simulink model "Cooperative_Quad_09_VelEst_02"  (R2017b)
settings: Solver=ode45  StartTime=0.0  StopTime=120  RelTol=1e-3  EnableMultiTasking=on
InitFcn:
  | Const_Vel_Est_02
values from neighbouring files (symbols this model uses):
  alpha = 1.0e-5    (= 1e-05)    [Cons_AMFC_Quad_New_01.m]    (also in Const_Vel_Est_02.m = 0.1; constant_Rev01_4Agents_10.m = 0.1; constant_Rev01_4Agents_9.m = 0.1)
  alpha_Slid = 0.01    [Cons_AMFC_Quad_New_01.m]    (also in Const_Vel_Est_02.m)
  AN = [     0 1 0 0 ... (first row only)    [Const_Vel_Est_02.m]    (also in constant_Rev01_4Agents_10.m; constant_Rev01_4Agents_9.m)
  B = 1e+0*eye(n)    [Cons_AMFC_Quad_New_01.m]    (also in Const_Vel_Est_02.m = 1e0*eye(n); constant_Rev01_4Agents_10.m = 1e0*eye(n); constant_Rev01_4Agents_9.m = 1e0*eye(n))
  BBT_inv = ((B'*B)^(-1))*B'    [Cons_AMFC_Quad_New_01.m]    (also in Const_Vel_Est_02.m; constant_Rev01_4Agents_10.m; constant_Rev01_4Agents_9.m)
  BN = [     1 0 0 0 ... (first row only)    [Const_Vel_Est_02.m]    (also in constant_Rev01_4Agents_10.m; constant_Rev01_4Agents_9.m)
  epsilon_struct = struct('data',epsilon_InitVal)    [Const_Vel_Est_02.m]    (also in constant_Rev01_4Agents_10.m; constant_Rev01_4Agents_9.m)
  g = 9.81    [Const_Vel_Est_02.m]    (also in Swing2d_01_const.m; constant_Rev01_4Agents_10.m; constant_Rev01_4Agents_9.m)
  gamma_0 = 1e-0*diag([1e-3*ones(3,1);1e-0*ones(3,1)])    [Cons_AMFC_Quad_New_01.m]    (also in Const_Vel_Est_02.m = 1e-1*diag([1e-3*ones(3,1);1e-0*ones(3,1)]); constant_Rev01_4Agents_10.m = 1e+1*diag([1e-3*ones(3,1);1e-0*ones(3,1)]); constant_Rev01_4Agents_9.m = 1e+1*diag([1e-3*ones(6,1);1e-0*ones(6,1)]))
  gamma_1 = 1e+2*diag([1e-3*ones(3,1);1e-0*ones(3,1)])    [Cons_AMFC_Quad_New_01.m]    (also in Const_Vel_Est_02.m; constant_Rev01_4Agents_10.m = 1e+3*diag([1e-3*ones(3,1);1e0*ones(3,1)]); constant_Rev01_4Agents_9.m = 1e+3*diag([1e-3*ones(6,1);1e0*ones(6,1)]))
  H = L + BN    [Const_Vel_Est_02.m]    (also in constant_Rev01_4Agents_10.m; constant_Rev01_4Agents_9.m)
  J = 1.2416e-3 * diag([1 1 2])    [Cons_AMFC_Quad_New_01.m]    (also in Const_Vel_Est_02.m = 1.2416e-3 * diag([1 1 2],0); constant_Rev01_4Agents_10.m = 1.2416e-3 * diag([1 1 2],0); constant_Rev01_4Agents_9.m = 1.2416e-3 * diag([1 1 2],0))
  k1 = 10    [Cons_AMFC_Quad_New_01.m]    (also in Const_Vel_Est_02.m = 1; constant_Rev01_4Agents_10.m = 1; constant_Rev01_4Agents_9.m = 1)
  k1o = 1000    [Cons_AMFC_Quad_New_01.m]    (also in Const_Vel_Est_02.m)
  k2 = 0.1    [Cons_AMFC_Quad_New_01.m]    (also in Const_Vel_Est_02.m; constant_Rev01_4Agents_10.m = 1; constant_Rev01_4Agents_9.m = 1)
  k2o = 100    [Cons_AMFC_Quad_New_01.m]    (also in Const_Vel_Est_02.m)
  Ka = 0.01    [Cons_AMFC_Quad_New_01.m]    (also in Const_Vel_Est_02.m; constant_Rev01_4Agents_10.m; constant_Rev01_4Agents_9.m)
  Kd = 0.01    [Cons_AMFC_Quad_New_01.m]    (also in Const_Vel_Est_02.m; constant_Rev01_4Agents_10.m; constant_Rev01_4Agents_9.m)
  Kf = 1.0e-5    (= 1e-05)    [Cons_AMFC_Quad_New_01.m]    (also in Const_Vel_Est_02.m; constant_Rev01_4Agents_10.m; constant_Rev01_4Agents_9.m)
  Kt = 0.0435 * Kf    (= 4.35e-07)    [Cons_AMFC_Quad_New_01.m]    (also in Const_Vel_Est_02.m = 1e-07; constant_Rev01_4Agents_10.m = 1e-07; constant_Rev01_4Agents_9.m = 1e-07)
  Lq = 0.2    [Const_Vel_Est_02.m]    (also in constant_Rev01_4Agents_10.m; constant_Rev01_4Agents_9.m)
  m = 6    [Cons_AMFC_Quad_New_01.m]    (also in Const_Vel_Est_02.m; Swing2d_01_const.m = 1)
  M = 2.95    [Cons_AMFC_Quad_New_01.m]    (also in Const_Vel_Est_02.m = 2; constant_Rev01_4Agents_10.m = 2; constant_Rev01_4Agents_9.m = 2)
  Mb_P = Mb_val_P*ones(np,1)    [Const_Vel_Est_02.m]
  Mb_V = Mb_val_V*ones(np,1)    [Const_Vel_Est_02.m]
  Mu_P = 10    [Const_Vel_Est_02.m]
  Mu_V = 10    [Const_Vel_Est_02.m]
  n = 6    [Cons_AMFC_Quad_New_01.m]    (also in Const_Vel_Est_02.m; constant_Rev01_4Agents_10.m; constant_Rev01_4Agents_9.m = 12)
  N = 4    [Const_Vel_Est_02.m]    (also in constant_Rev01_4Agents_10.m; constant_Rev01_4Agents_9.m)
  n0 = 3    [Const_Vel_Est_02.m]    (also in constant_Rev01_4Agents_10.m; constant_Rev01_4Agents_9.m)
  np = 2    [Const_Vel_Est_02.m]
  Observer_Gain = 100    [Const_Vel_Est_02.m]    (also in constant_Rev01_4Agents_10.m; constant_Rev01_4Agents_9.m)
  Observer_Gain1 = 100    [Const_Vel_Est_02.m]    (also in constant_Rev01_4Agents_10.m = 10; constant_Rev01_4Agents_9.m = 10)
  Q = 1e-1*eye(n)    [Cons_AMFC_Quad_New_01.m]    (also in Const_Vel_Est_02.m = 1e-2*eye(n); constant_Rev01_4Agents_10.m = 1e-3*eye(n); constant_Rev01_4Agents_9.m = 1e-3*eye(n))
  R = 1e+0*eye(m)    [Cons_AMFC_Quad_New_01.m]    (also in Const_Vel_Est_02.m = 1e-0*eye(n); constant_Rev01_4Agents_10.m = 1e-0*eye(n); constant_Rev01_4Agents_9.m = 1e-0*eye(n))
  rho_0 = 1e-1    (= 0.1)    [Cons_AMFC_Quad_New_01.m]    (also in Const_Vel_Est_02.m; constant_Rev01_4Agents_10.m = 10; constant_Rev01_4Agents_9.m = 10)
  rho_1 = 1e-0    (= 1)    [Cons_AMFC_Quad_New_01.m]    (also in Const_Vel_Est_02.m; constant_Rev01_4Agents_10.m = 0.1; constant_Rev01_4Agents_9.m = 0.1)
  T_struct = struct('data',T_InitVal)    [Const_Vel_Est_02.m]    (also in constant_Rev01_4Agents_10.m; constant_Rev01_4Agents_9.m)
  U_dot0_M = U_dot0_m*ones(n0,1)    [Const_Vel_Est_02.m]    (also in constant_Rev01_4Agents_10.m; constant_Rev01_4Agents_9.m)
  Upsilon_M = Upsilon_m*ones(n0,1)    [Const_Vel_Est_02.m]    (also in constant_Rev01_4Agents_10.m; constant_Rev01_4Agents_9.m)
undefined symbols (not defined in the file or in its folder): sigbuilder_block
(part 1 of 5)
settings Model: SimulationMode=rapid-accelerator  Creator=hp  LastModifiedBy=ali.safaei
settings DataIOCC: LimitDataPoints=on  SaveFormat=Array
settings OptimizationCC: LifeSpan=inf
settings DebuggingCC: UnderspecifiedInitializationDetection=Classic  MergeDetectMultiDrivingBlocksExec=none  SFUnexpectedBacktrackingDiag=warning  SFNoUnconditionalDefaultTransitionDiag=warning  SFExecutionAtInitializationDiag=none
settings HardwareCC: ProdBitPerPointer=32  ProdBitPerSizeT=32  ProdBitPerPtrDiffT=32  ProdLargestAtomicFloat=None  ProdIntDivRoundTo=Undefined  ProdEndianess=Unspecified  ProdWordSize=32  ProdHWDeviceType=32-bit Generic
settings ModelReferenceCC: PropagateSignalLabelsOutOfModel=off
settings CodeAppCC: StateflowObjectComments=on
settings GRTTargetCC: TargetLangStandard=C89/C90 (ANSI)  GeneratePreprocessorConditionals=Disable all
settings ConfigComp: CovMetricSettings=dw  CovHtmlReporting=on  CovSaveCumulativeToWorkspaceVar=on  CovSaveSingleToWorkspaceVar=on  CovExternalEMLEnable=off

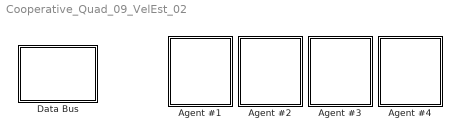
== system Cooperative_Quad_09_VelEst_02 ==
  Agent #1 : Subsystem
  Agent #2 : Subsystem
  Agent #3 : Subsystem
  Agent #4 : Subsystem
  "Data Bus " : Subsystem

== system Cooperative_Quad_09_VelEst_02/Agent #1 ==
  Agent # : Constant
  Constant1 : Constant  Value=zeros(2,1)
  Constant2 : Constant  Value=zeros(2,1)
  Decenteralized Cooperaive Controller #1 : Subsystem
  Mux1 : Mux
  Mux2 : Mux
  Plant #1 : Subsystem
  Relative estimations-1 : Subsystem
  tag scope: Acc1_XY=global, P_rel01_XY=global, P_rel1_XY=global, Pos1_XY=global, Pos1_Z=global, V_rel01_XY=global, V_rel1_XY=global, Vel1_XY=global, x1=global
  wires:
  Agent #/1 -> Decenteralized Cooperaive Controller #1/1(Agent #)
  Plant #1/1(X) -> [x1]
  Decenteralized Cooperaive Controller #1/1(u1) -> Plant #1/1(U)
  Plant #1/2(P_XY) -> Relative estimations-1/1(P_local_XY), [Pos1_XY]
  Plant #1/3(A_XY) -> [Acc1_XY], Relative estimations-1/2(A_local_XY)
  Mux1/1 -> [P_rel1_XY]
  Relative estimations-1/7(P10_est) -> [P_rel01_XY]
  Constant2/1 -> Mux1/1
  Relative estimations-1/8(V10_est) -> [V_rel01_XY]
  Constant1/1 -> Mux2/1
  Mux2/1 -> [V_rel1_XY]
  Relative estimations-1/1(P12_est) -> Mux1/2
  Relative estimations-1/3(P13_est) -> Mux1/3
  Relative estimations-1/5(P14_est) -> Mux1/4
  Relative estimations-1/2(V12_est) -> Mux2/2
  Relative estimations-1/4(V13_est) -> Mux2/3
  Relative estimations-1/6(V14_est) -> Mux2/4
  Plant #1/4(P_Z) -> [Pos1_Z]
  Plant #1/5(V_XY) -> [Vel1_XY]

== system Cooperative_Quad_09_VelEst_02/Agent #2 ==
  Agent # : Constant  Value=2
  Constant1 : Constant  Value=zeros(2,1)
  Constant2 : Constant  Value=zeros(2,1)
  Decenteralized Cooperaive Controller #2 : Subsystem
  Mux1 : Mux
  Mux2 : Mux
  Plant #2 : Subsystem
  Relative estimations-2 : Subsystem
  tag scope: Acc2_XY=global, P_rel02_XY=global, P_rel2_XY=global, Pos2_XY=global, Pos2_Z=global, V_rel02_XY=global, V_rel2_XY=global, Vel2_XY=global, x2=global
  wires:
  Plant #2/4(P_Z) -> [Pos2_Z]
  Relative estimations-2/6(V24_est) -> Mux2/4
  Relative estimations-2/4(V23_est) -> Mux2/3
  Relative estimations-2/2(V21_est) -> Mux2/2
  Relative estimations-2/5(P24_est) -> Mux1/4
  Relative estimations-2/3(P23_est) -> Mux1/3
  Relative estimations-2/1(P21_est) -> Mux1/2
  Mux2/1 -> [V_rel2_XY]
  Constant1/1 -> Mux2/1
  Relative estimations-2/8(V20_est) -> [V_rel02_XY]
  Constant2/1 -> Mux1/1
  Relative estimations-2/7(P20_est) -> [P_rel02_XY]
  Mux1/1 -> [P_rel2_XY]
  Plant #2/3(A_XY) -> [Acc2_XY], Relative estimations-2/2(A_local_XY)
  Plant #2/2(P_XY) -> [Pos2_XY], Relative estimations-2/1(P_local_XY)
  Decenteralized Cooperaive Controller #2/1(u2) -> Plant #2/1(U)
  Plant #2/1(X) -> [x2]
  Agent #/1 -> Decenteralized Cooperaive Controller #2/1(Agent #)
  Plant #2/5(V_XY) -> [Vel2_XY]

== system Cooperative_Quad_09_VelEst_02/Agent #3 ==
  Agent # : Constant  Value=3
  Constant1 : Constant  Value=zeros(2,1)
  Constant2 : Constant  Value=zeros(2,1)
  Decenteralized Cooperaive Controller #3 : Subsystem
  Mux1 : Mux
  Mux2 : Mux
  Plant #3 : Subsystem
  Relative estimations-3 : Subsystem
  tag scope: Acc3_XY=global, P_rel03_XY=global, P_rel3_XY=global, Pos3_XY=global, Pos3_Z=global, V_rel03_XY=global, V_rel3_XY=global, Vel3_XY=global, x3=global
  wires:
  Agent #/1 -> Decenteralized Cooperaive Controller #3/1(Agent #)
  Plant #3/1(X) -> [x3]
  Decenteralized Cooperaive Controller #3/1(u3) -> Plant #3/1(U)
  Plant #3/2(P_XY) -> Relative estimations-3/1(P_local_XY), [Pos3_XY]
  Plant #3/3(A_XY) -> [Acc3_XY], Relative estimations-3/2(A_local_XY)
  Mux1/1 -> [P_rel3_XY]
  Relative estimations-3/7(P30_est) -> [P_rel03_XY]
  Constant2/1 -> Mux1/1
  Relative estimations-3/8(V30_est) -> [V_rel03_XY]
  Constant1/1 -> Mux2/1
  Mux2/1 -> [V_rel3_XY]
  Relative estimations-3/1(P31_est) -> Mux1/2
  Relative estimations-3/3(P32_est) -> Mux1/3
  Relative estimations-3/5(P34_est) -> Mux1/4
  Relative estimations-3/2(V31_est) -> Mux2/2
  Relative estimations-3/4(V32_est) -> Mux2/3
  Relative estimations-3/6(V34_est) -> Mux2/4
  Plant #3/4(P_Z) -> [Pos3_Z]
  Plant #3/5(V_XY) -> [Vel3_XY]

== system Cooperative_Quad_09_VelEst_02/Agent #4 ==
  Agent # : Constant  Value=4
  Constant1 : Constant  Value=zeros(2,1)
  Constant2 : Constant  Value=zeros(2,1)
  Decenteralized Cooperaive Controller #4 : Subsystem
  Mux1 : Mux
  Mux2 : Mux
  Plant #4 : Subsystem
  Relative estimations-4 : Subsystem
  tag scope: Acc4_XY=global, P_rel04_XY=global, P_rel4_XY=global, Pos4_XY=global, Pos4_Z=global, V_rel04_XY=global, V_rel4_XY=global, Vel4_XY=global, x4=global
  wires:
  Plant #4/4(P_Z) -> [Pos4_Z]
  Relative estimations-4/6(V43_est) -> Mux2/4
  Relative estimations-4/4(V42_est) -> Mux2/3
  Relative estimations-4/2(V41_est) -> Mux2/2
  Relative estimations-4/5(P43_est) -> Mux1/4
  Relative estimations-4/3(P42_est) -> Mux1/3
  Relative estimations-4/1(P41_est) -> Mux1/2
  Mux2/1 -> [V_rel4_XY]
  Constant1/1 -> Mux2/1
  Relative estimations-4/8(V40_est) -> [V_rel04_XY]
  Constant2/1 -> Mux1/1
  Relative estimations-4/7(P40_est) -> [P_rel04_XY]
  Mux1/1 -> [P_rel4_XY]
  Plant #4/3(A_XY) -> Relative estimations-4/2(A_local_XY), [Acc4_XY]
  Plant #4/2(P_XY) -> Relative estimations-4/1(P_local_XY), [Pos4_XY]
  Decenteralized Cooperaive Controller #4/1(u4) -> Plant #4/1(U)
  Plant #4/1(X) -> [x4]
  Agent #/1 -> Decenteralized Cooperaive Controller #4/1(Agent #)
  Plant #4/5(V_XY) -> [Vel4_XY]

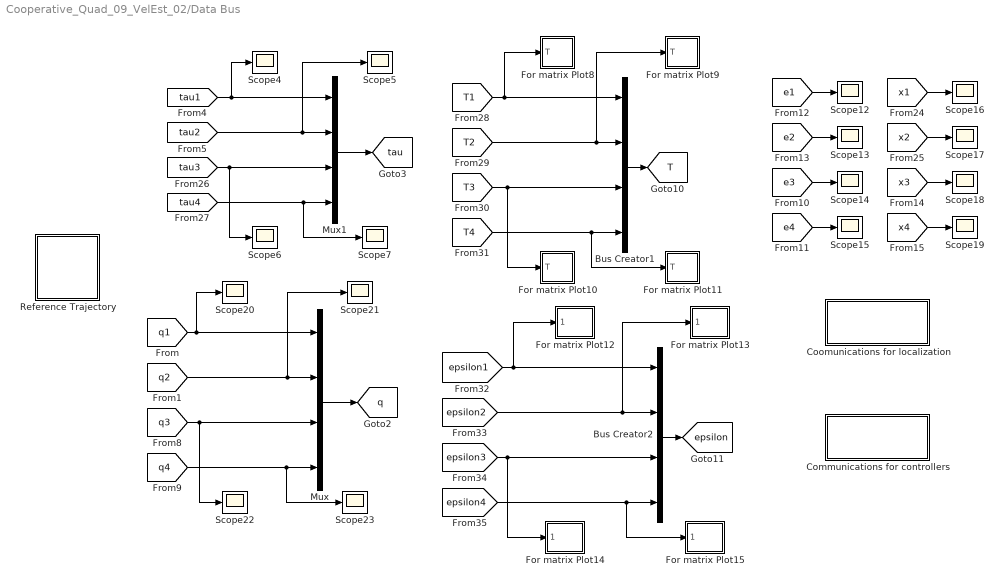
== system Cooperative_Quad_09_VelEst_02/Data Bus  ==
  Bus Creator1 : BusCreator  Inputs=4  OutDataTypeStr=Bus: T_bus
  Bus Creator2 : BusCreator  Inputs=4  OutDataTypeStr=Bus: epsilon_bus
  Communications for controllers : Subsystem
  Coomunications for localization : Subsystem
  For matrix Plot10 : Subsystem
  For matrix Plot11 : Subsystem
  For matrix Plot12 : Subsystem
  For matrix Plot13 : Subsystem
  For matrix Plot14 : Subsystem
  For matrix Plot15 : Subsystem
  For matrix Plot8 : Subsystem
  For matrix Plot9 : Subsystem
  Mux : Mux
  Mux1 : Mux
  Reference Trajectory : Subsystem
  Scope{4..7,12..23} (16 alike) : Scope
  tag scope: T=global, epsilon=global, q=global, tau=global
  wires:
  [q2] -> Scope21/1, Mux/2
  [tau1] -> Scope4/1, Mux1/1
  [tau2] -> Scope5/1, Mux1/2
  Mux1/1 -> [tau]
  [q1] -> Scope20/1, Mux/1
  Mux/1 -> [q]
  [e2] -> Scope13/1
  [e1] -> Scope12/1
  [x1] -> Scope16/1
  [q4] -> Scope23/1, Mux/4
  [q3] -> Scope22/1, Mux/3
  [e3] -> Scope14/1
  [e4] -> Scope15/1
  [x3] -> Scope18/1
  [x4] -> Scope19/1
  [tau3] -> Scope6/1, Mux1/3
  [tau4] -> Scope7/1, Mux1/4
  [T2] -> For matrix Plot9/1(T), Bus Creator1/2
  [T1] -> For matrix Plot8/1(T), Bus Creator1/1
  Bus Creator1/1 -> [T]
  [T3] -> For matrix Plot10/1(T), Bus Creator1/3
  [T4] -> For matrix Plot11/1(T), Bus Creator1/4
  [epsilon2] -> For matrix Plot13/1(epsilon), Bus Creator2/2
  [epsilon1] -> For matrix Plot12/1(epsilon), Bus Creator2/1
  Bus Creator2/1 -> [epsilon]
  [epsilon3] -> For matrix Plot14/1(epsilon), Bus Creator2/3
  [epsilon4] -> For matrix Plot15/1(epsilon), Bus Creator2/4
  [x2] -> Scope17/1

== system Cooperative_Quad_09_VelEst_02/Agent #1/Decenteralized Cooperaive Controller #1 ==
  Agent # : Inport
  Ali-1 : Subsystem
  "Computing xd-1 " : MATLAB Function  TreatAsAtomicUnit=on
  Cooperative Observers for X-1 : Subsystem
  Cooperative Observers for Xd-1 : Subsystem
  Mux : Mux  Inputs=2
  Subsystem : Subsystem
  Sum2 : Sum  Inputs=|+-
  u1 : Outport
  tag scope: e1=global
  wires:
  Agent #/1 -> "Computing xd-1 "/3(Agent_Num), Cooperative Observers for Xd-1/1(Agent No.), Cooperative Observers for X-1/1(Agent No.)
  Ali-1/1(u) -> u1/1
  "Computing xd-1 "/1(xd) -> Subsystem/1(In1)
  Subsystem/1(Out1) -> Sum2/1, Ali-1/2(xd)
  Cooperative Observers for Xd-1/1(q1) -> "Computing xd-1 "/1(q_i)
  Cooperative Observers for Xd-1/2(T1) -> "Computing xd-1 "/2(T_i)
  Cooperative Observers for X-1/1(X_est1) -> Ali-1/1(x)
  Sum2/1 -> [e1]
  [Pos1_XY] -> Mux/1
  Mux/1 -> Sum2/2
  [Pos1_Z] -> Mux/2

== system Cooperative_Quad_09_VelEst_02/Agent #1/Plant #1 ==
  U : Inport
  Clock : Clock
  Demux1 : Demux
  Integrator : Integrator  InitialCondition=zeros(2*n,1)
  MATLAB Function : MATLAB Function  TreatAsAtomicUnit=on
  Memory : Memory  InitialCondition=zeros(np,1)
  Memory1 : Memory  InitialCondition=zeros(np,1)
  Memory2 : Memory
  Memory3 : Memory  InitialCondition=zeros(np,1)
  X : Outport
  P_XY : Outport  Port=2
  A_XY : Outport  Port=3
  P_Z : Outport  Port=4
  V_XY : Outport  Port=5
  wires:
  MATLAB Function/1(DX) -> Integrator/1
  Integrator/1 -> MATLAB Function/1(X), X/1
  Demux1/1 -> MATLAB Function/2(u1)
  Demux1/2 -> MATLAB Function/3(u2)
  Demux1/3 -> MATLAB Function/4(u3)
  Demux1/4 -> MATLAB Function/5(u4)
  U/1 -> Demux1/1
  Clock/1 -> MATLAB Function/6(t)
  MATLAB Function/2(Pos_XY) -> Memory/1
  Memory/1 -> P_XY/1
  MATLAB Function/5(Acc_XY) -> Memory1/1
  Memory1/1 -> A_XY/1
  Memory2/1 -> P_Z/1
  MATLAB Function/3(Pos_Z) -> Memory2/1
  Memory3/1 -> V_XY/1
  MATLAB Function/4(Vel_XY) -> Memory3/1

== system Cooperative_Quad_09_VelEst_02/Agent #1/Relative estimations-1 ==
  P_local_XY : Inport
  A_local_XY : Inport  Port=2
  Rel_10 : Subsystem
  Rel_12 : Subsystem
  Rel_13 : Subsystem
  Rel_14 : Subsystem
  P12_est : Outport
  V12_est : Outport  Port=2
  P13_est : Outport  Port=3
  V13_est : Outport  Port=4
  P14_est : Outport  Port=5
  V14_est : Outport  Port=6
  P10_est : Outport  Port=7
  V10_est : Outport  Port=8
  wires:
  Rel_12/1(P_rel_12) -> P12_est/1
  Rel_12/2(V_rel_12) -> V12_est/1
  Rel_13/2(V_rel_13) -> V13_est/1
  Rel_13/1(P_rel_13) -> P13_est/1
  Rel_14/1(P_rel_14) -> P14_est/1
  Rel_14/2(V_rel_14) -> V14_est/1
  Rel_10/2(V_rel_10) -> V10_est/1
  Rel_10/1(P_rel_10) -> P10_est/1
  A_local_XY/1 -> Rel_10/1(A_local_XY), Rel_13/1(A_local_XY), Rel_14/1(A_local_XY), Rel_12/1(A_local_XY)
  P_local_XY/1 -> Rel_12/2(P_local_XY), Rel_14/2(P_local_XY), Rel_13/2(P_local_XY), Rel_10/2(P_local_XY)

== system Cooperative_Quad_09_VelEst_02/Agent #2/Decenteralized Cooperaive Controller #2 ==
  Agent # : Inport
  Ali-2 : Subsystem
  "Computing xd-2 " : MATLAB Function  TreatAsAtomicUnit=on
  Cooperative Observers for X-2 : Subsystem
  Cooperative Observers for Xd-2 : Subsystem
  Mux : Mux  Inputs=2
  Subsystem : Subsystem
  Sum2 : Sum  Inputs=|+-
  u2 : Outport
  tag scope: e2=global
  wires:
  Cooperative Observers for X-2/1(X_est2) -> Ali-2/1(x)
  Cooperative Observers for Xd-2/2(T2) -> "Computing xd-2 "/2(T_i)
  Cooperative Observers for Xd-2/1(q2) -> "Computing xd-2 "/1(q_i)
  "Computing xd-2 "/1(xd) -> Subsystem/1(In1)
  Ali-2/1(u) -> u2/1
  Agent #/1 -> Cooperative Observers for Xd-2/1(Agent No.), Cooperative Observers for X-2/1(Agent No.), "Computing xd-2 "/3(Agent_Num)
  Mux/1 -> Sum2/2
  [Pos2_XY] -> Mux/1
  Sum2/1 -> [e2]
  [Pos2_Z] -> Mux/2
  Subsystem/1(Out1) -> Sum2/1, Ali-2/2(xd)

== system Cooperative_Quad_09_VelEst_02/Agent #2/Plant #2 ==
  U : Inport
  Clock : Clock
  Demux1 : Demux
  Integrator : Integrator  InitialCondition=zeros(2*n,1)
  MATLAB Function : MATLAB Function  TreatAsAtomicUnit=on
  Memory : Memory  InitialCondition=zeros(np,1)
  Memory1 : Memory  InitialCondition=zeros(np,1)
  Memory2 : Memory
  Memory3 : Memory  InitialCondition=zeros(np,1)
  X : Outport
  P_XY : Outport  Port=2
  A_XY : Outport  Port=3
  P_Z : Outport  Port=4
  V_XY : Outport  Port=5
  wires:
  MATLAB Function/1(DX) -> Integrator/1
  Integrator/1 -> MATLAB Function/1(X), X/1
  Demux1/1 -> MATLAB Function/2(u1)
  Demux1/2 -> MATLAB Function/3(u2)
  Demux1/3 -> MATLAB Function/4(u3)
  Demux1/4 -> MATLAB Function/5(u4)
  U/1 -> Demux1/1
  Clock/1 -> MATLAB Function/6(t)
  MATLAB Function/2(Pos_XY) -> Memory/1
  Memory/1 -> P_XY/1
  MATLAB Function/5(Acc_XY) -> Memory1/1
  Memory1/1 -> A_XY/1
  Memory2/1 -> P_Z/1
  MATLAB Function/3(Pos_Z) -> Memory2/1
  Memory3/1 -> V_XY/1
  MATLAB Function/4(Vel_XY) -> Memory3/1

== system Cooperative_Quad_09_VelEst_02/Agent #2/Relative estimations-2 ==
  P_local_XY : Inport
  A_local_XY : Inport  Port=2
  Rel_20 : Subsystem
  Rel_21 : Subsystem
  Rel_23 : Subsystem
  Rel_24 : Subsystem
  P21_est : Outport
  V21_est : Outport  Port=2
  P23_est : Outport  Port=3
  V23_est : Outport  Port=4
  P24_est : Outport  Port=5
  V24_est : Outport  Port=6
  P20_est : Outport  Port=7
  V20_est : Outport  Port=8
  wires:
  P_local_XY/1 -> Rel_20/2(P_local_XY), Rel_23/2(P_local_XY), Rel_24/2(P_local_XY), Rel_21/2(P_local_XY)
  A_local_XY/1 -> Rel_21/1(A_local_XY), Rel_24/1(A_local_XY), Rel_23/1(A_local_XY), Rel_20/1(A_local_XY)
  Rel_20/1(P_rel_20) -> P20_est/1
  Rel_20/2(V_rel_20) -> V20_est/1
  Rel_24/2(V_rel_24) -> V24_est/1
  Rel_24/1(P_rel_24) -> P24_est/1
  Rel_23/1(P_rel_23) -> P23_est/1
  Rel_23/2(V_rel_23) -> V23_est/1
  Rel_21/2(V_rel_21) -> V21_est/1
  Rel_21/1(P_rel_21) -> P21_est/1

== system Cooperative_Quad_09_VelEst_02/Agent #3/Decenteralized Cooperaive Controller #3 ==
  Agent # : Inport
  Ali-3 : Subsystem
  "Computing xd-3 " : MATLAB Function  TreatAsAtomicUnit=on
  Cooperative Observers for X-3 : Subsystem
  Cooperative Observers for Xd-3 : Subsystem
  Mux : Mux  Inputs=2
  Subsystem : Subsystem
  Sum2 : Sum  Inputs=|+-
  u3 : Outport
  tag scope: e3=global
  wires:
  Agent #/1 -> "Computing xd-3 "/3(Agent_Num), Cooperative Observers for X-3/1(Agent No.), Cooperative Observers for Xd-3/1(Agent No.)
  Ali-3/1(u) -> u3/1
  "Computing xd-3 "/1(xd) -> Subsystem/1(In1)
  Subsystem/1(Out1) -> Sum2/1, Ali-3/2(xd)
  Cooperative Observers for Xd-3/1(q3) -> "Computing xd-3 "/1(q_i)
  Cooperative Observers for Xd-3/2(T3) -> "Computing xd-3 "/2(T_i)
  Cooperative Observers for X-3/1(X_est3) -> Ali-3/1(x)
  Mux/1 -> Sum2/2
  [Pos3_XY] -> Mux/1
  Sum2/1 -> [e3]
  [Pos3_Z] -> Mux/2

== system Cooperative_Quad_09_VelEst_02/Agent #3/Plant #3 ==
  U : Inport
  Clock : Clock
  Demux1 : Demux
  Integrator : Integrator  InitialCondition=zeros(2*n,1)
  MATLAB Function : MATLAB Function  TreatAsAtomicUnit=on
  Memory : Memory  InitialCondition=zeros(np,1)
  Memory1 : Memory  InitialCondition=zeros(np,1)
  Memory2 : Memory
  Memory3 : Memory  InitialCondition=zeros(np,1)
  X : Outport
  P_XY : Outport  Port=2
  A_XY : Outport  Port=3
  P_Z : Outport  Port=4
  V_XY : Outport  Port=5
  wires:
  MATLAB Function/1(DX) -> Integrator/1
  Integrator/1 -> MATLAB Function/1(X), X/1
  Demux1/1 -> MATLAB Function/2(u1)
  Demux1/2 -> MATLAB Function/3(u2)
  Demux1/3 -> MATLAB Function/4(u3)
  Demux1/4 -> MATLAB Function/5(u4)
  U/1 -> Demux1/1
  Clock/1 -> MATLAB Function/6(t)
  MATLAB Function/2(Pos_XY) -> Memory/1
  Memory/1 -> P_XY/1
  MATLAB Function/5(Acc_XY) -> Memory1/1
  Memory1/1 -> A_XY/1
  Memory2/1 -> P_Z/1
  MATLAB Function/3(Pos_Z) -> Memory2/1
  Memory3/1 -> V_XY/1
  MATLAB Function/4(Vel_XY) -> Memory3/1

== system Cooperative_Quad_09_VelEst_02/Agent #3/Relative estimations-3 ==
  P_local_XY : Inport
  A_local_XY : Inport  Port=2
  Rel_30 : Subsystem
  Rel_31 : Subsystem
  Rel_32 : Subsystem
  Rel_34 : Subsystem
  P31_est : Outport
  V31_est : Outport  Port=2
  P32_est : Outport  Port=3
  V32_est : Outport  Port=4
  P34_est : Outport  Port=5
  V34_est : Outport  Port=6
  P30_est : Outport  Port=7
  V30_est : Outport  Port=8
  wires:
  Rel_31/1(P_rel_31) -> P31_est/1
  Rel_31/2(V_rel_31) -> V31_est/1
  Rel_32/2(V_rel_32) -> V32_est/1
  Rel_32/1(P_rel_32) -> P32_est/1
  Rel_34/1(P_rel_34) -> P34_est/1
  Rel_34/2(V_rel_34) -> V34_est/1
  Rel_30/2(V_rel_30) -> V30_est/1
  Rel_30/1(P_rel_30) -> P30_est/1
  A_local_XY/1 -> Rel_30/1(A_local_XY), Rel_32/1(A_local_XY), Rel_34/1(A_local_XY), Rel_31/1(A_local_XY)
  P_local_XY/1 -> Rel_31/2(P_local_XY), Rel_34/2(P_local_XY), Rel_32/2(P_local_XY), Rel_30/2(P_local_XY)

== system Cooperative_Quad_09_VelEst_02/Agent #4/Decenteralized Cooperaive Controller #4 ==
  Agent # : Inport
  Ali-4 : Subsystem
  "Computing xd-4 " : MATLAB Function  TreatAsAtomicUnit=on
  Cooperative Observers for X-4 : Subsystem
  Cooperative Observers for Xd-4 : Subsystem
  Mux : Mux  Inputs=2
  Subsystem : Subsystem
  Sum2 : Sum  Inputs=|+-
  u4 : Outport
  tag scope: e4=global
  wires:
  Cooperative Observers for X-4/1(X_est4) -> Ali-4/1(x)
  Cooperative Observers for Xd-4/2(T4) -> "Computing xd-4 "/2(T_i)
  Cooperative Observers for Xd-4/1(q4) -> "Computing xd-4 "/1(q_i)
  Subsystem/1(Out1) -> Sum2/1, Ali-4/2(xd)
  "Computing xd-4 "/1(xd) -> Subsystem/1(In1)
  Ali-4/1(u) -> u4/1
  Agent #/1 -> Cooperative Observers for Xd-4/1(Agent No.), Cooperative Observers for X-4/1(Agent No.), "Computing xd-4 "/3(Agent_Num)
  Mux/1 -> Sum2/2
  [Pos4_XY] -> Mux/1
  Sum2/1 -> [e4]
  [Pos4_Z] -> Mux/2

== system Cooperative_Quad_09_VelEst_02/Agent #4/Plant #4 ==
  U : Inport
  Clock : Clock
  Demux1 : Demux
  Integrator : Integrator  InitialCondition=zeros(2*n,1)
  MATLAB Function : MATLAB Function  TreatAsAtomicUnit=on
  Memory : Memory  InitialCondition=zeros(np,1)
  Memory1 : Memory  InitialCondition=zeros(np,1)
  Memory2 : Memory
  Memory3 : Memory  InitialCondition=zeros(np,1)
  X : Outport
  P_XY : Outport  Port=2
  A_XY : Outport  Port=3
  P_Z : Outport  Port=4
  V_XY : Outport  Port=5
  wires:
  MATLAB Function/1(DX) -> Integrator/1
  Integrator/1 -> MATLAB Function/1(X), X/1
  Demux1/1 -> MATLAB Function/2(u1)
  Demux1/2 -> MATLAB Function/3(u2)
  Demux1/3 -> MATLAB Function/4(u3)
  Demux1/4 -> MATLAB Function/5(u4)
  U/1 -> Demux1/1
  Clock/1 -> MATLAB Function/6(t)
  MATLAB Function/2(Pos_XY) -> Memory/1
  Memory/1 -> P_XY/1
  MATLAB Function/5(Acc_XY) -> Memory1/1
  Memory1/1 -> A_XY/1
  Memory2/1 -> P_Z/1
  MATLAB Function/3(Pos_Z) -> Memory2/1
  Memory3/1 -> V_XY/1
  MATLAB Function/4(Vel_XY) -> Memory3/1

== system Cooperative_Quad_09_VelEst_02/Agent #4/Relative estimations-4 ==
  P_local_XY : Inport
  A_local_XY : Inport  Port=2
  Rel_40 : Subsystem
  Rel_41 : Subsystem
  Rel_42 : Subsystem
  Rel_43 : Subsystem
  P41_est : Outport
  V41_est : Outport  Port=2
  P42_est : Outport  Port=3
  V42_est : Outport  Port=4
  P43_est : Outport  Port=5
  V43_est : Outport  Port=6
  P40_est : Outport  Port=7
  V40_est : Outport  Port=8
  wires:
  P_local_XY/1 -> Rel_40/2(P_local_XY), Rel_42/2(P_local_XY), Rel_43/2(P_local_XY), Rel_41/2(P_local_XY)
  A_local_XY/1 -> Rel_41/1(A_local_XY), Rel_43/1(A_local_XY), Rel_42/1(A_local_XY), Rel_40/1(A_local_XY)
  Rel_40/1(P_rel_40) -> P40_est/1
  Rel_40/2(V_rel_40) -> V40_est/1
  Rel_43/2(V_rel_43) -> V43_est/1
  Rel_43/1(P_rel_43) -> P43_est/1
  Rel_42/1(P_rel_42) -> P42_est/1
  Rel_42/2(V_rel_42) -> V42_est/1
  Rel_41/2(V_rel_41) -> V41_est/1
  Rel_41/1(P_rel_41) -> P41_est/1

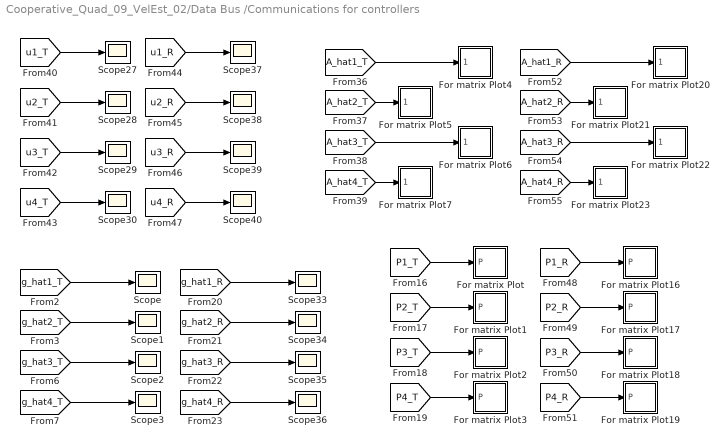
== system Cooperative_Quad_09_VelEst_02/Data Bus /Communications for controllers ==
  For matrix Plot : Subsystem
  For matrix Plot1 : Subsystem
  For matrix Plot16 : Subsystem
  For matrix Plot17 : Subsystem
  For matrix Plot18 : Subsystem
  For matrix Plot19 : Subsystem
  For matrix Plot2 : Subsystem
  For matrix Plot20 : Subsystem
  For matrix Plot21 : Subsystem
  For matrix Plot22 : Subsystem
  For matrix Plot23 : Subsystem
  For matrix Plot3 : Subsystem
  For matrix Plot4 : Subsystem
  For matrix Plot5 : Subsystem
  For matrix Plot6 : Subsystem
  For matrix Plot7 : Subsystem
  Scope{,1..3,27..30,33..40} (16 alike) : Scope
  wires:
  [A_hat4_T] -> For matrix Plot7/1(A_hat)
  [A_hat3_T] -> For matrix Plot6/1(A_hat)
  [A_hat2_T] -> For matrix Plot5/1(A_hat)
  [A_hat2_R] -> For matrix Plot21/1(A_hat)
  [A_hat1_R] -> For matrix Plot20/1(A_hat)
  [A_hat3_R] -> For matrix Plot22/1(A_hat)
  [A_hat4_R] -> For matrix Plot23/1(A_hat)
  [A_hat1_T] -> For matrix Plot4/1(A_hat)
  [u4_R] -> Scope40/1
  [u1_T] -> Scope27/1
  [u1_R] -> Scope37/1
  [u3_T] -> Scope29/1
  [u3_R] -> Scope39/1
  [u4_T] -> Scope30/1
  [u2_R] -> Scope38/1
  [u2_T] -> Scope28/1
  [g_hat3_T] -> Scope2/1
  [g_hat1_T] -> Scope/1
  [g_hat4_T] -> Scope3/1
  [g_hat2_T] -> Scope1/1
  [g_hat1_R] -> Scope33/1
  [g_hat4_R] -> Scope36/1
  [g_hat2_R] -> Scope34/1
  [g_hat3_R] -> Scope35/1
  [P4_R] -> For matrix Plot19/1(P)
  [P4_T] -> For matrix Plot3/1(P)
  [P1_T] -> For matrix Plot/1(P)
  [P3_R] -> For matrix Plot18/1(P)
  [P3_T] -> For matrix Plot2/1(P)
  [P1_R] -> For matrix Plot16/1(P)
  [P2_T] -> For matrix Plot1/1(P)
  [P2_R] -> For matrix Plot17/1(P)

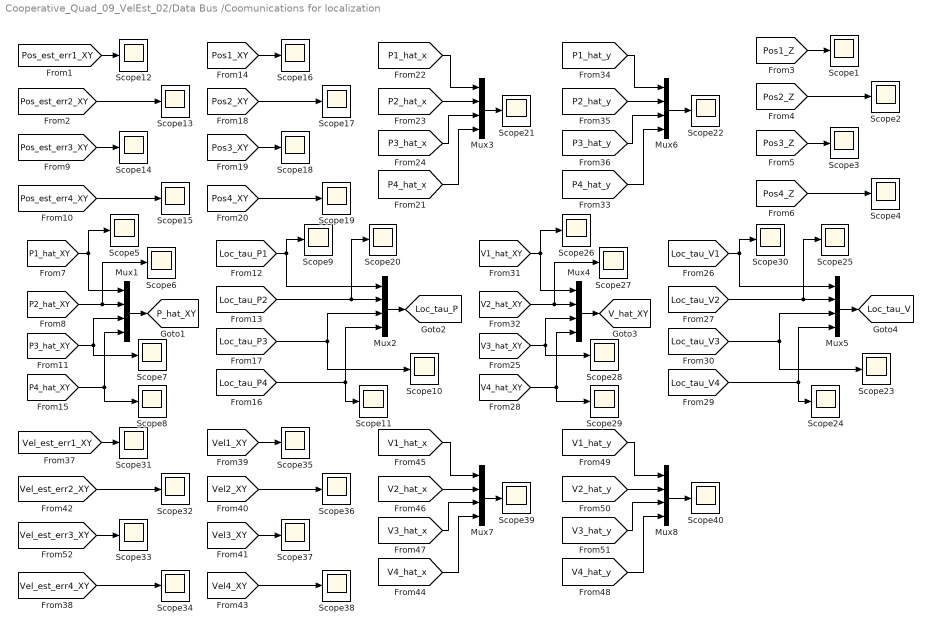
== system Cooperative_Quad_09_VelEst_02/Data Bus /Coomunications for localization ==
  Mux{1..8} (8 alike) : Mux
  Scope{1..40} (40 alike) : Scope
  tag scope: Loc_tau_P=global, Loc_tau_V=global, P_hat_XY=global, V_hat_XY=global
  wires:
  Mux6/1 -> Scope22/1
  [P4_hat_y] -> Mux6/4
  Mux3/1 -> Scope21/1
  [P4_hat_x] -> Mux3/4
  [Pos2_XY] -> Scope17/1
  [Pos3_XY] -> Scope18/1
  [Pos1_XY] -> Scope16/1
  [Pos4_XY] -> Scope19/1
  [Pos_est_err3_XY] -> Scope14/1
  [Pos_est_err4_XY] -> Scope15/1
  [P3_hat_x] -> Mux3/3
  [P1_hat_y] -> Mux6/1
  [Pos_est_err1_XY] -> Scope12/1
  [P3_hat_y] -> Mux6/3
  [P2_hat_y] -> Mux6/2
  [Pos_est_err2_XY] -> Scope13/1
  [P1_hat_x] -> Mux3/1
  [P2_hat_x] -> Mux3/2
  [Pos4_Z] -> Scope4/1
  [Pos1_Z] -> Scope1/1
  [Pos3_Z] -> Scope3/1
  [Pos2_Z] -> Scope2/1
  [P4_hat_XY] -> Scope8/1, Mux1/4
  [Loc_tau_P1] -> Scope9/1, Mux2/1
  [Loc_tau_P4] -> Scope11/1, Mux2/4
  [Loc_tau_P2] -> Scope20/1, Mux2/2
  Mux2/1 -> [Loc_tau_P]
  [P3_hat_XY] -> Scope7/1, Mux1/3
  [P2_hat_XY] -> Scope6/1, Mux1/2
  [P1_hat_XY] -> Scope5/1, Mux1/1
  Mux1/1 -> [P_hat_XY]
  [Loc_tau_P3] -> Mux2/3, Scope10/1
  [Loc_tau_V3] -> Scope23/1, Mux5/3
  Mux4/1 -> [V_hat_XY]
  [V1_hat_XY] -> Mux4/1, Scope26/1
  [V2_hat_XY] -> Mux4/2, Scope27/1
  [V3_hat_XY] -> Mux4/3, Scope28/1
  Mux5/1 -> [Loc_tau_V]
  [Loc_tau_V2] -> Mux5/2, Scope25/1
  [Loc_tau_V4] -> Mux5/4, Scope24/1
  [Loc_tau_V1] -> Mux5/1, Scope30/1
  [V4_hat_XY] -> Mux4/4, Scope29/1
  [V2_hat_x] -> Mux7/2
  [V2_hat_y] -> Mux8/2
  [V3_hat_y] -> Mux8/3
  [V1_hat_y] -> Mux8/1
  [Vel_est_err1_XY] -> Scope31/1
  [V4_hat_x] -> Mux7/4
  Mux8/1 -> Scope40/1
  [Vel1_XY] -> Scope35/1
  [Vel3_XY] -> Scope37/1
  [Vel_est_err2_XY] -> Scope32/1
  Mux7/1 -> Scope39/1
  [V1_hat_x] -> Mux7/1
  [V4_hat_y] -> Mux8/4
  [V3_hat_x] -> Mux7/3
  [Vel_est_err3_XY] -> Scope33/1
  [Vel2_XY] -> Scope36/1
  [Vel_est_err4_XY] -> Scope34/1
  [Vel4_XY] -> Scope38/1

== system Cooperative_Quad_09_VelEst_02/Data Bus /For matrix Plot10 ==
  T : Inport
  MATLAB Function : MATLAB Function  TreatAsAtomicUnit=on
  Scope24 : Scope
  To Workspace : ToWorkspace  VariableName=T3  SaveFormat=Structure With Time  SampleTime=-1
  wires:
  T/1 -> MATLAB Function/1(u)
  MATLAB Function/1(y) -> Scope24/1, To Workspace/1

== system Cooperative_Quad_09_VelEst_02/Data Bus /For matrix Plot11 ==
  T : Inport
  MATLAB Function : MATLAB Function  TreatAsAtomicUnit=on
  Scope24 : Scope
  To Workspace : ToWorkspace  VariableName=T4  SaveFormat=Structure With Time  SampleTime=-1
  wires:
  MATLAB Function/1(y) -> Scope24/1, To Workspace/1
  T/1 -> MATLAB Function/1(u)

== system Cooperative_Quad_09_VelEst_02/Data Bus /For matrix Plot12 ==
  epsilon : Inport
  MATLAB Function : MATLAB Function  TreatAsAtomicUnit=on
  Scope24 : Scope
  To Workspace : ToWorkspace  VariableName=epsilon1  SaveFormat=Structure With Time  SampleTime=-1
  wires:
  epsilon/1 -> MATLAB Function/1(u)
  MATLAB Function/1(y) -> Scope24/1, To Workspace/1

== system Cooperative_Quad_09_VelEst_02/Data Bus /For matrix Plot13 ==
  epsilon : Inport
  MATLAB Function : MATLAB Function  TreatAsAtomicUnit=on
  Scope24 : Scope
  To Workspace : ToWorkspace  VariableName=epsilon2  SaveFormat=Structure With Time  SampleTime=-1
  wires:
  MATLAB Function/1(y) -> Scope24/1, To Workspace/1
  epsilon/1 -> MATLAB Function/1(u)

== system Cooperative_Quad_09_VelEst_02/Data Bus /For matrix Plot14 ==
  epsilon : Inport
  MATLAB Function : MATLAB Function  TreatAsAtomicUnit=on
  Scope24 : Scope
  To Workspace : ToWorkspace  VariableName=epsilon3  SaveFormat=Structure With Time  SampleTime=-1
  wires:
  MATLAB Function/1(y) -> Scope24/1, To Workspace/1
  epsilon/1 -> MATLAB Function/1(u)

== system Cooperative_Quad_09_VelEst_02/Data Bus /For matrix Plot15 ==
  epsilon : Inport
  MATLAB Function : MATLAB Function  TreatAsAtomicUnit=on
  Scope24 : Scope
  To Workspace : ToWorkspace  VariableName=epsilon4  SaveFormat=Structure With Time  SampleTime=-1
  wires:
  epsilon/1 -> MATLAB Function/1(u)
  MATLAB Function/1(y) -> Scope24/1, To Workspace/1

== system Cooperative_Quad_09_VelEst_02/Data Bus /For matrix Plot8 ==
  T : Inport
  MATLAB Function : MATLAB Function  TreatAsAtomicUnit=on
  Scope24 : Scope
  To Workspace : ToWorkspace  VariableName=T1  SaveFormat=Structure With Time  SampleTime=-1
  wires:
  MATLAB Function/1(y) -> Scope24/1, To Workspace/1
  T/1 -> MATLAB Function/1(u)

== system Cooperative_Quad_09_VelEst_02/Data Bus /For matrix Plot9 ==
  T : Inport
  MATLAB Function : MATLAB Function  TreatAsAtomicUnit=on
  Scope24 : Scope
  To Workspace : ToWorkspace  VariableName=T2  SaveFormat=Structure With Time  SampleTime=-1
  wires:
  T/1 -> MATLAB Function/1(u)
  MATLAB Function/1(y) -> Scope24/1, To Workspace/1

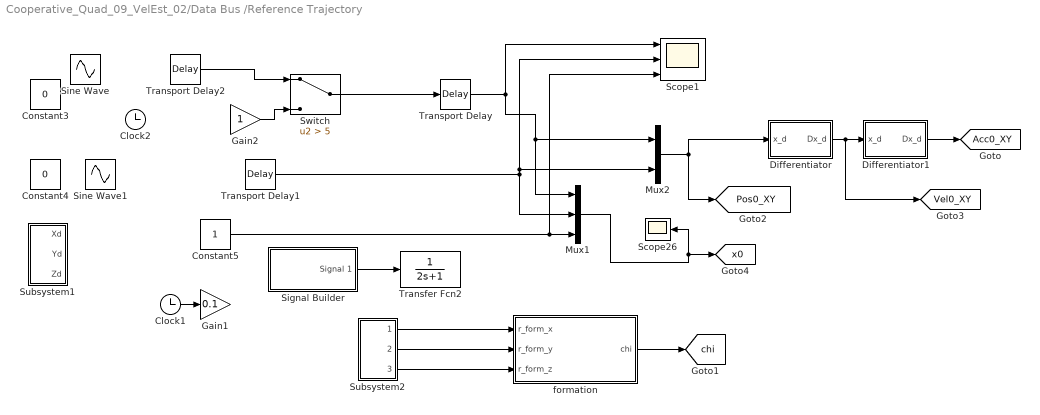
== system Cooperative_Quad_09_VelEst_02/Data Bus /Reference Trajectory ==
  Clock1 : Clock
  Clock2 : Clock
  Constant3 : Constant  Value=0
  Constant4 : Constant  Value=0
  Constant5 : Constant
  Differentiator : Subsystem
  Differentiator1 : Subsystem
  Gain1 : Gain  Gain=0.1
  Gain2 : Gain
  Mux1 : Mux  Inputs=3
  Mux2 : Mux  Inputs=2
  Scope1 : Scope  NumInputPorts=3
  Scope26 : Scope
  Signal Builder : Subsystem  Tag=STV Subsys  LoadFcn=sigbuilder_block('load');  StartFcn=sigbuilder_block('start');  StopFcn=sigbuilder_block('stop');  ClipboardFcn=sigbuilder_block('clipboard');  mask(Sigbuilder block){tuvar=[0:10]}
      mask help: Simulink:masks:SigbuilderBlock_MD
      mask init:
      | if ~strcmp(get_param(bdroot(gcbh),'SimulationStatus'),'stopped') tuvar = sigbuilder_block('maskInit'); end
      settings: CopyFcn=sigbuilder_block('copy');  DeleteFcn=sigbuilder_block('delete');  ModelCloseFcn=sigbuilder_block('modelClose');  PreSaveFcn=sigbuilder_block('preSave');  PauseFcn=sigbuilder_block('pause');  ContinueFcn=sigbuilder_block('continue');  NameChangeFcn=sigbuilder_block('namechange');  OpenFcn=sigbuilder_block('open',[437.25 117.75 550.5 394.5 ]);  CloseFcn=sigbuilder_block('close');
      mask Display: plot(0, 0, 100, 100,[2, 2, 32, 32, 2], [68, 8, 8, 68, 68],[32, 2], [38, 38], [32, 19, 2],[53, 60, 44], [32, 17, 17, 2],[16, 16, 31, 31]);txt = getActiveGroup(gcbh);text(2, 100, txt,'verticalAlignment', 'top');
  Sine Wave : Sin  Amplitude=5  Frequency=0.2  Phase=pi/2  SampleTime=0
  Sine Wave1 : Sin  Amplitude=5  Frequency=0.2  SampleTime=0
  Subsystem1 : Subsystem
  Subsystem2 : Subsystem
  Switch : Switch  Criteria=u2 > Threshold  Threshold=5
  Transfer Fcn2 : TransferFcn  Denominator=[2 1]
  Transport Delay : TransportDelay  DelayTime=5
  Transport Delay1 : TransportDelay  DelayTime=10
  Transport Delay2 : TransportDelay  DelayTime=5
  formation : MATLAB Function  TreatAsAtomicUnit=on
  tag scope: Acc0_XY=global, Pos0_XY=global, Vel0_XY=global, chi=global, x0=global
  wires:
  Clock1/1 -> Gain1/1
  Signal Builder/1(Signal 1) -> Transfer Fcn2/1
  Constant5/1 -> Scope1/3, Mux1/3
  ? -> Transport Delay1/1
  Transport Delay1/1 -> Mux1/2, Mux2/2, Scope1/2
  Transport Delay/1 -> Mux2/1, Mux1/1, Scope1/1
  formation/1(chi) -> [chi]
  Subsystem2/1(form_x) -> formation/1(r_form_x)
  Subsystem2/2(form_y) -> formation/2(r_form_y)
  Subsystem2/3(form_z) -> formation/3(r_form_z)
  Switch/1 -> Transport Delay/1
  ? -> Switch/2, Gain2/1
  ? -> Transport Delay2/1
  Gain2/1 -> Switch/3
  Transport Delay2/1 -> Switch/1
  Differentiator1/1(Dx_d) -> [Acc0_XY]
  Mux1/1 -> [x0], Scope26/1
  Mux2/1 -> [Pos0_XY], Differentiator/1(x_d)
  Differentiator/1(Dx_d) -> Differentiator1/1(x_d), [Vel0_XY]

== system Cooperative_Quad_09_VelEst_02/Agent #1/Decenteralized Cooperaive Controller #1/Ali-1 ==
  x : Inport
  xd : Inport  Port=2
  Controller interpreter-1 : MATLAB Function  TreatAsAtomicUnit=on
  Controller interpreter1-1 : MATLAB Function  TreatAsAtomicUnit=on
  Rotational-1 : Subsystem
  Translational-1 : Subsystem
  u : Outport
  wires:
  Controller interpreter-1/2(PHI_d) -> Rotational-1/1(x_rd)
  Rotational-1/1(ur) -> Controller interpreter1-1/2(ur)
  Controller interpreter1-1/1(u) -> u/1
  Controller interpreter-1/1(u0) -> Controller interpreter1-1/1(u0t)
  xd/1 -> Translational-1/1(x_td)
  x/1 -> Rotational-1/2(X), Translational-1/2(x_t)
  Translational-1/1(ut) -> Controller interpreter-1/1(u)

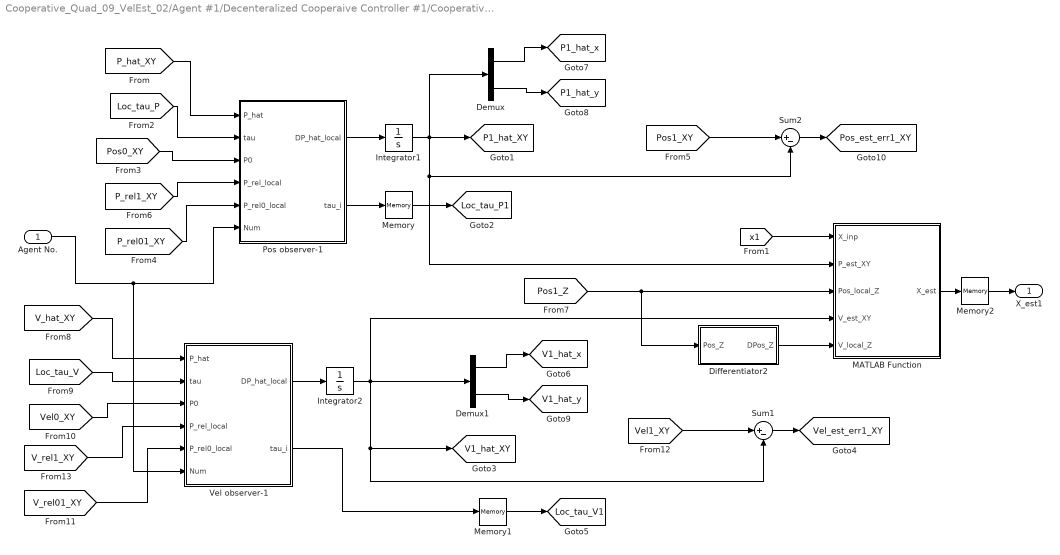
== system Cooperative_Quad_09_VelEst_02/Agent #1/Decenteralized Cooperaive Controller #1/Cooperative Observers for X-1 ==
  Agent No. : Inport
  Demux : Demux  Outputs=2
  Demux1 : Demux  Outputs=2
  Differentiator2 : Subsystem
  Integrator1 : Integrator  InitialCondition=zeros(np,1)
  Integrator2 : Integrator  InitialCondition=zeros(np,1)
  MATLAB Function : MATLAB Function  TreatAsAtomicUnit=on
  Memory : Memory  InitialCondition=zeros(np,1)
  Memory1 : Memory  InitialCondition=zeros(np,1)
  Memory2 : Memory  InitialCondition=zeros(2*n,1)
  Pos observer-1 : MATLAB Function  TreatAsAtomicUnit=on
  Sum1 : Sum  Inputs=|+-
  Sum2 : Sum  Inputs=|+-
  Vel observer-1 : MATLAB Function  TreatAsAtomicUnit=on
  X_est1 : Outport
  tag scope: Loc_tau_P1=global, Loc_tau_V1=global, P1_hat_XY=global, P1_hat_x=global, P1_hat_y=global, Pos_est_err1_XY=global, V1_hat_XY=global, V1_hat_x=global, V1_hat_y=global, Vel_est_err1_XY=global
  wires:
  [Pos1_XY] -> Sum2/1
  [Loc_tau_P] -> Pos observer-1/2(tau)
  [P_rel01_XY] -> Pos observer-1/5(P_rel0_local)
  Pos observer-1/1(DP_hat_local) -> Integrator1/1
  Pos observer-1/2(tau_i) -> Memory/1
  Demux/1 -> [P1_hat_x]
  Memory/1 -> [Loc_tau_P1]
  [Pos0_XY] -> Pos observer-1/3(P0)
  [P_hat_XY] -> Pos observer-1/1(P_hat)
  Sum2/1 -> [Pos_est_err1_XY]
  [P_rel1_XY] -> Pos observer-1/4(P_rel_local)
  Demux/2 -> [P1_hat_y]
  Integrator1/1 -> Sum2/2, MATLAB Function/2(P_est_XY), Demux/1, [P1_hat_XY]
  Agent No./1 -> Vel observer-1/6(Num), Pos observer-1/6(Num)
  MATLAB Function/1(X_est) -> Memory2/1
  [x1] -> MATLAB Function/1(X_inp)
  [Pos1_Z] -> Differentiator2/1(Pos_Z), MATLAB Function/3(Pos_local_Z)
  Differentiator2/1(DPos_Z) -> MATLAB Function/5(V_local_Z)
  [Vel1_XY] -> Sum1/1
  Integrator2/1 -> Sum1/2, [V1_hat_XY], Demux1/1, MATLAB Function/4(V_est_XY)
  Demux1/2 -> [V1_hat_y]
  [V_rel1_XY] -> Vel observer-1/4(P_rel_local)
  [Loc_tau_V] -> Vel observer-1/2(tau)
  [V_hat_XY] -> Vel observer-1/1(P_hat)
  Sum1/1 -> [Vel_est_err1_XY]
  [V_rel01_XY] -> Vel observer-1/5(P_rel0_local)
  [Vel0_XY] -> Vel observer-1/3(P0)
  Demux1/1 -> [V1_hat_x]
  Memory1/1 -> [Loc_tau_V1]
  Vel observer-1/2(tau_i) -> Memory1/1
  Vel observer-1/1(DP_hat_local) -> Integrator2/1
  Memory2/1 -> X_est1/1

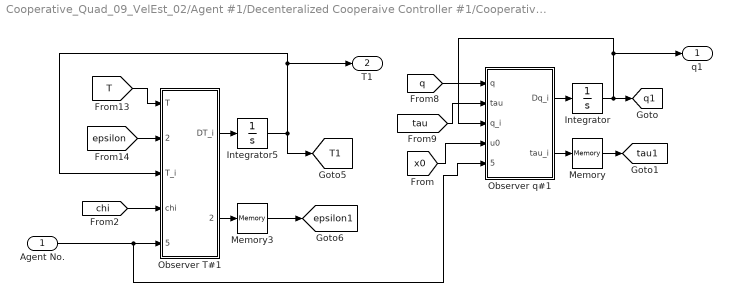
== system Cooperative_Quad_09_VelEst_02/Agent #1/Decenteralized Cooperaive Controller #1/Cooperative Observers for Xd-1 ==
  Agent No. : Inport
  Integrator : Integrator  InitialCondition=zeros(n0,1)
  Integrator5 : Integrator  InitialCondition=zeros(N+1,n0)
  Memory : Memory  InitialCondition=zeros(n0,1)
  Memory3 : Memory  InitialCondition=zeros(N+1,n0)
  Observer T#1 : MATLAB Function  TreatAsAtomicUnit=on
  Observer q#1 : MATLAB Function  TreatAsAtomicUnit=on
  q1 : Outport
  T1 : Outport  Port=2
  tag scope: T1=global, epsilon1=global, q1=global, tau1=global
  wires:
  [chi] -> Observer T#1/4(chi)
  [epsilon] -> Observer T#1/2(epsilon)
  Observer T#1/1(DT_i) -> Integrator5/1
  [T] -> Observer T#1/1(T)
  Observer T#1/2(epsilon_i) -> Memory3/1
  Observer q#1/1(Dq_i) -> Integrator/1
  Memory/1 -> [tau1]
  [x0] -> Observer q#1/4(u0)
  Observer q#1/2(tau_i) -> Memory/1
  Agent No./1 -> Observer q#1/5(Agent_Num), Observer T#1/5(Agent_Num)
  Integrator5/1 -> [T1], T1/1, Observer T#1/3(T_i)
  [q] -> Observer q#1/1(q)
  Integrator/1 -> [q1], q1/1, Observer q#1/3(q_i)
  [tau] -> Observer q#1/2(tau)
  Memory3/1 -> [epsilon1]

== system Cooperative_Quad_09_VelEst_02/Agent #1/Decenteralized Cooperaive Controller #1/Subsystem ==
  In1 : Inport
  Demux : Demux  Outputs=3
  Mux : Mux  Inputs=3
  Transport Delay1 : TransportDelay  DelayTime=5
  Transport Delay2 : TransportDelay  DelayTime=5
  Out1 : Outport
  wires:
  In1/1 -> Demux/1
  Demux/1 -> Transport Delay1/1
  Demux/2 -> Transport Delay2/1
  Mux/1 -> Out1/1
  Transport Delay2/1 -> Mux/2
  Transport Delay1/1 -> Mux/1
  Demux/3 -> Mux/3

== system Cooperative_Quad_09_VelEst_02/Agent #1/Relative estimations-1/Rel_10 ==
  A_local_XY : Inport
  P_local_XY : Inport  Port=2
  Differentiator1 : Subsystem
  Integrator1 : Integrator  InitialCondition=zeros(2,1)
  Integrator2 : Integrator  InitialCondition=zeros(2,1)
  Relative estimation1 : MATLAB Function  TreatAsAtomicUnit=on
  Relative estimation2 : MATLAB Function  TreatAsAtomicUnit=on
  Relative measurements1 : MATLAB Function  TreatAsAtomicUnit=on
  Sum : Sum  Inputs=|+-
  P_rel_10 : Outport
  V_rel_10 : Outport  Port=2
  wires:
  Sum/1 -> Relative estimation2/1(A_rel)
  [Acc0_XY] -> Sum/2
  [Pos0_XY] -> Relative measurements1/1(P_other)
  Differentiator1/1(Dx_d) -> Relative estimation2/2(dv)
  Relative estimation2/1(DV_est) -> Integrator1/1
  Relative estimation1/1(DP_est) -> Integrator2/1
  P_local_XY/1 -> Relative measurements1/2(P_local)
  A_local_XY/1 -> Sum/1
  Integrator1/1 -> Relative estimation1/1(V_rel), V_rel_10/1, Relative estimation2/3(V_est)
  Relative measurements1/1(d) -> Relative estimation1/2(dp), Differentiator1/1(x_d)
  Integrator2/1 -> Relative estimation1/3(P_est), P_rel_10/1

== system Cooperative_Quad_09_VelEst_02/Agent #1/Relative estimations-1/Rel_12 ==
  A_local_XY : Inport
  P_local_XY : Inport  Port=2
  Differentiator1 : Subsystem
  Integrator1 : Integrator  InitialCondition=zeros(2,1)
  Integrator2 : Integrator  InitialCondition=zeros(2,1)
  Relative estimation1 : MATLAB Function  TreatAsAtomicUnit=on
  Relative estimation2 : MATLAB Function  TreatAsAtomicUnit=on
  Relative measurements1 : MATLAB Function  TreatAsAtomicUnit=on
  Sum : Sum  Inputs=|+-
  P_rel_12 : Outport
  V_rel_12 : Outport  Port=2
  wires:
  Integrator2/1 -> P_rel_12/1, Relative estimation1/3(P_est)
  Relative measurements1/1(d) -> Differentiator1/1(x_d), Relative estimation1/2(dp)
  Integrator1/1 -> Relative estimation2/3(V_est), V_rel_12/1, Relative estimation1/1(V_rel)
  A_local_XY/1 -> Sum/1
  P_local_XY/1 -> Relative measurements1/2(P_local)
  Relative estimation1/1(DP_est) -> Integrator2/1
  Relative estimation2/1(DV_est) -> Integrator1/1
  Differentiator1/1(Dx_d) -> Relative estimation2/2(dv)
  [Pos2_XY] -> Relative measurements1/1(P_other)
  [Acc2_XY] -> Sum/2
  Sum/1 -> Relative estimation2/1(A_rel)

== system Cooperative_Quad_09_VelEst_02/Agent #1/Relative estimations-1/Rel_13 ==
  A_local_XY : Inport
  P_local_XY : Inport  Port=2
  Differentiator1 : Subsystem
  Integrator1 : Integrator  InitialCondition=zeros(2,1)
  Integrator2 : Integrator  InitialCondition=zeros(2,1)
  Relative estimation1 : MATLAB Function  TreatAsAtomicUnit=on
  Relative estimation2 : MATLAB Function  TreatAsAtomicUnit=on
  Relative measurements1 : MATLAB Function  TreatAsAtomicUnit=on
  Sum : Sum  Inputs=|+-
  P_rel_13 : Outport
  V_rel_13 : Outport  Port=2
  wires:
  Sum/1 -> Relative estimation2/1(A_rel)
  [Acc3_XY] -> Sum/2
  [Pos3_XY] -> Relative measurements1/1(P_other)
  Differentiator1/1(Dx_d) -> Relative estimation2/2(dv)
  Relative estimation2/1(DV_est) -> Integrator1/1
  Relative estimation1/1(DP_est) -> Integrator2/1
  P_local_XY/1 -> Relative measurements1/2(P_local)
  A_local_XY/1 -> Sum/1
  Integrator1/1 -> Relative estimation2/3(V_est), Relative estimation1/1(V_rel), V_rel_13/1
  Relative measurements1/1(d) -> Relative estimation1/2(dp), Differentiator1/1(x_d)
  Integrator2/1 -> Relative estimation1/3(P_est), P_rel_13/1

== system Cooperative_Quad_09_VelEst_02/Agent #1/Relative estimations-1/Rel_14 ==
  A_local_XY : Inport
  P_local_XY : Inport  Port=2
  Differentiator1 : Subsystem
  Integrator1 : Integrator  InitialCondition=zeros(2,1)
  Integrator2 : Integrator  InitialCondition=zeros(2,1)
  Relative estimation1 : MATLAB Function  TreatAsAtomicUnit=on
  Relative estimation2 : MATLAB Function  TreatAsAtomicUnit=on
  Relative measurements1 : MATLAB Function  TreatAsAtomicUnit=on
  Sum : Sum  Inputs=|+-
  P_rel_14 : Outport
  V_rel_14 : Outport  Port=2
  wires:
  Integrator2/1 -> P_rel_14/1, Relative estimation1/3(P_est)
  Relative measurements1/1(d) -> Differentiator1/1(x_d), Relative estimation1/2(dp)
  Integrator1/1 -> Relative estimation2/3(V_est), V_rel_14/1, Relative estimation1/1(V_rel)
  A_local_XY/1 -> Sum/1
  P_local_XY/1 -> Relative measurements1/2(P_local)
  Relative estimation1/1(DP_est) -> Integrator2/1
  Relative estimation2/1(DV_est) -> Integrator1/1
  Differentiator1/1(Dx_d) -> Relative estimation2/2(dv)
  [Pos4_XY] -> Relative measurements1/1(P_other)
  [Acc4_XY] -> Sum/2
  Sum/1 -> Relative estimation2/1(A_rel)

== system Cooperative_Quad_09_VelEst_02/Agent #2/Decenteralized Cooperaive Controller #2/Ali-2 ==
  x : Inport
  xd : Inport  Port=2
  Controller interpreter-2 : MATLAB Function  TreatAsAtomicUnit=on
  Controller interpreter1-2 : MATLAB Function  TreatAsAtomicUnit=on
  Rotational-2 : Subsystem
  Translational-2 : Subsystem
  u : Outport
  wires:
  Translational-2/1(ut) -> Controller interpreter-2/1(u)
  x/1 -> Translational-2/2(x_t), Rotational-2/2(X)
  xd/1 -> Translational-2/1(x_td)
  Controller interpreter-2/1(u0) -> Controller interpreter1-2/1(u0t)
  Controller interpreter1-2/1(u) -> u/1
  Rotational-2/1(ur) -> Controller interpreter1-2/2(ur)
  Controller interpreter-2/2(PHI_d) -> Rotational-2/1(x_rd)

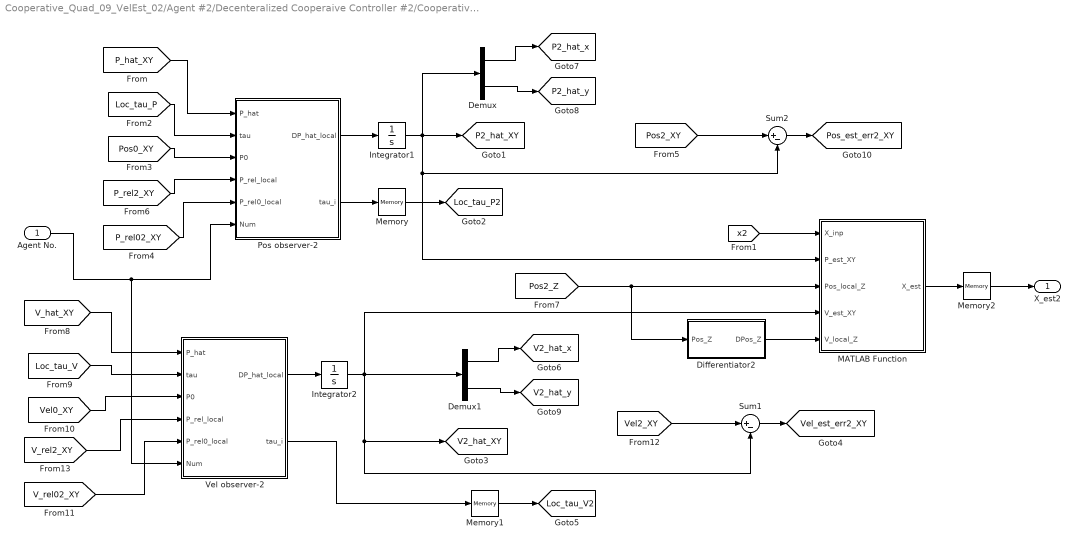
== system Cooperative_Quad_09_VelEst_02/Agent #2/Decenteralized Cooperaive Controller #2/Cooperative Observers for X-2 ==
  Agent No. : Inport
  Demux : Demux  Outputs=2
  Demux1 : Demux  Outputs=2
  Differentiator2 : Subsystem
  Integrator1 : Integrator  InitialCondition=zeros(np,1)
  Integrator2 : Integrator  InitialCondition=zeros(np,1)
  MATLAB Function : MATLAB Function  TreatAsAtomicUnit=on
  Memory : Memory  InitialCondition=zeros(np,1)
  Memory1 : Memory  InitialCondition=zeros(np,1)
  Memory2 : Memory  InitialCondition=zeros(2*n,1)
  Pos observer-2 : MATLAB Function  TreatAsAtomicUnit=on
  Sum1 : Sum  Inputs=|+-
  Sum2 : Sum  Inputs=|+-
  Vel observer-2 : MATLAB Function  TreatAsAtomicUnit=on
  X_est2 : Outport
  tag scope: Loc_tau_P2=global, Loc_tau_V2=global, P2_hat_XY=global, P2_hat_x=global, P2_hat_y=global, Pos_est_err2_XY=global, V2_hat_XY=global, V2_hat_x=global, V2_hat_y=global, Vel_est_err2_XY=global
  wires:
  Vel observer-2/1(DP_hat_local) -> Integrator2/1
  Vel observer-2/2(tau_i) -> Memory1/1
  Memory1/1 -> [Loc_tau_V2]
  Demux1/1 -> [V2_hat_x]
  [Vel0_XY] -> Vel observer-2/3(P0)
  [V_rel02_XY] -> Vel observer-2/5(P_rel0_local)
  Sum1/1 -> [Vel_est_err2_XY]
  [V_hat_XY] -> Vel observer-2/1(P_hat)
  [Loc_tau_V] -> Vel observer-2/2(tau)
  [V_rel2_XY] -> Vel observer-2/4(P_rel_local)
  Demux1/2 -> [V2_hat_y]
  Integrator2/1 -> MATLAB Function/4(V_est_XY), Demux1/1, [V2_hat_XY], Sum1/2
  [Vel2_XY] -> Sum1/1
  Differentiator2/1(DPos_Z) -> MATLAB Function/5(V_local_Z)
  [Pos2_Z] -> MATLAB Function/3(Pos_local_Z), Differentiator2/1(Pos_Z)
  [x2] -> MATLAB Function/1(X_inp)
  MATLAB Function/1(X_est) -> Memory2/1
  Agent No./1 -> Pos observer-2/6(Num), Vel observer-2/6(Num)
  Integrator1/1 -> [P2_hat_XY], Demux/1, MATLAB Function/2(P_est_XY), Sum2/2
  Demux/2 -> [P2_hat_y]
  [P_rel2_XY] -> Pos observer-2/4(P_rel_local)
  Sum2/1 -> [Pos_est_err2_XY]
  [P_hat_XY] -> Pos observer-2/1(P_hat)
  [Pos0_XY] -> Pos observer-2/3(P0)
  Memory/1 -> [Loc_tau_P2]
  Demux/1 -> [P2_hat_x]
  Pos observer-2/2(tau_i) -> Memory/1
  Pos observer-2/1(DP_hat_local) -> Integrator1/1
  [P_rel02_XY] -> Pos observer-2/5(P_rel0_local)
  [Loc_tau_P] -> Pos observer-2/2(tau)
  [Pos2_XY] -> Sum2/1
  Memory2/1 -> X_est2/1

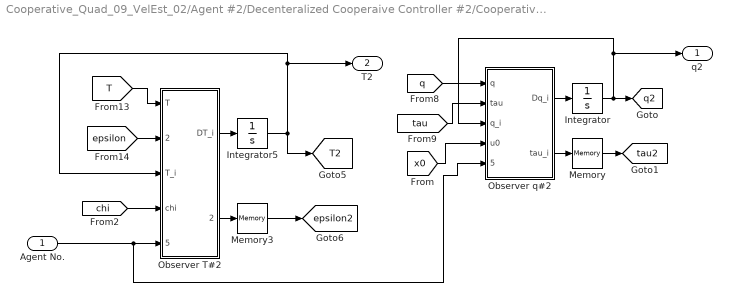
== system Cooperative_Quad_09_VelEst_02/Agent #2/Decenteralized Cooperaive Controller #2/Cooperative Observers for Xd-2 ==
  Agent No. : Inport
  Integrator : Integrator  InitialCondition=zeros(n0,1)
  Integrator5 : Integrator  InitialCondition=zeros(N+1,n0)
  Memory : Memory  InitialCondition=zeros(n0,1)
  Memory3 : Memory  InitialCondition=zeros(N+1,n0)
  Observer T#2 : MATLAB Function  TreatAsAtomicUnit=on
  Observer q#2 : MATLAB Function  TreatAsAtomicUnit=on
  q2 : Outport
  T2 : Outport  Port=2
  tag scope: T2=global, epsilon2=global, q2=global, tau2=global
  wires:
  Memory3/1 -> [epsilon2]
  [tau] -> Observer q#2/2(tau)
  Integrator/1 -> Observer q#2/3(q_i), q2/1, [q2]
  [q] -> Observer q#2/1(q)
  Integrator5/1 -> Observer T#2/3(T_i), T2/1, [T2]
  Agent No./1 -> Observer T#2/5(Agent_Num), Observer q#2/5(Agent_Num)
  Observer q#2/2(tau_i) -> Memory/1
  [x0] -> Observer q#2/4(u0)
  Memory/1 -> [tau2]
  Observer q#2/1(Dq_i) -> Integrator/1
  Observer T#2/2(epsilon_i) -> Memory3/1
  [T] -> Observer T#2/1(T)
  Observer T#2/1(DT_i) -> Integrator5/1
  [epsilon] -> Observer T#2/2(epsilon)
  [chi] -> Observer T#2/4(chi)

== system Cooperative_Quad_09_VelEst_02/Agent #2/Decenteralized Cooperaive Controller #2/Subsystem ==
  In1 : Inport
  Demux : Demux  Outputs=3
  Mux : Mux  Inputs=3
  Transport Delay1 : TransportDelay  DelayTime=5
  Transport Delay2 : TransportDelay  DelayTime=5
  Out1 : Outport
  wires:
  Demux/3 -> Mux/3
  Transport Delay1/1 -> Mux/1
  Transport Delay2/1 -> Mux/2
  Mux/1 -> Out1/1
  Demux/2 -> Transport Delay2/1
  Demux/1 -> Transport Delay1/1
  In1/1 -> Demux/1

== system Cooperative_Quad_09_VelEst_02/Agent #2/Relative estimations-2/Rel_20 ==
  A_local_XY : Inport
  P_local_XY : Inport  Port=2
  Differentiator1 : Subsystem
  Integrator1 : Integrator  InitialCondition=zeros(2,1)
  Integrator2 : Integrator  InitialCondition=zeros(2,1)
  Relative estimation1 : MATLAB Function  TreatAsAtomicUnit=on
  Relative estimation2 : MATLAB Function  TreatAsAtomicUnit=on
  Relative measurements1 : MATLAB Function  TreatAsAtomicUnit=on
  Sum : Sum  Inputs=|+-
  P_rel_20 : Outport
  V_rel_20 : Outport  Port=2
  wires:
  Integrator2/1 -> P_rel_20/1, Relative estimation1/3(P_est)
  Relative measurements1/1(d) -> Differentiator1/1(x_d), Relative estimation1/2(dp)
  Integrator1/1 -> Relative estimation2/3(V_est), V_rel_20/1, Relative estimation1/1(V_rel)
  A_local_XY/1 -> Sum/1
  P_local_XY/1 -> Relative measurements1/2(P_local)
  Relative estimation1/1(DP_est) -> Integrator2/1
  Relative estimation2/1(DV_est) -> Integrator1/1
  Differentiator1/1(Dx_d) -> Relative estimation2/2(dv)
  [Pos0_XY] -> Relative measurements1/1(P_other)
  [Acc0_XY] -> Sum/2
  Sum/1 -> Relative estimation2/1(A_rel)
